simulink model "ADConverter_sim_2020"  (R2020b)
settings: Solver=ode4  StartTime=0.0  StopTime=20  FixedStep=0.05  RelTol=1e-3
settings Model: Creator=005274  LastModifiedBy=005274

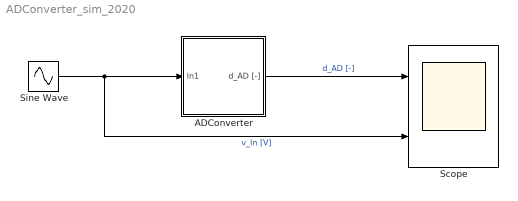
== system ADConverter_sim_2020 ==
  ADConverter : Subsystem  mask{n=10, V_max=5, V_min=0}
      mask prompts: n "Resolution : n bit"
  Scope : Scope  NumInputPorts=2
  Sine Wave : Sin  Amplitude=10  Frequency=2*pi*0.1  SampleTime=0
  wires:
  Sine Wave/1 -> Scope/2, ADConverter/1(In1)  "v_In [V]"
  ADConverter/1(d_AD [-]) -> Scope/1  "d_AD [-]"

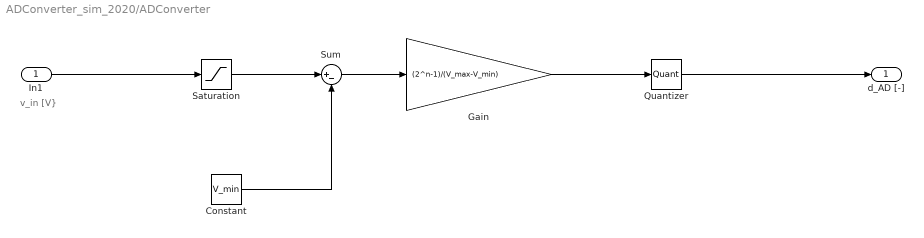
== system ADConverter_sim_2020/ADConverter ==
  note: v_in [V}
  In1 : Inport
  Constant : Constant  Value=V_min
  Gain : Gain  Gain=(2^n-1)/(V_max-V_min)
  Quantizer : Quantizer
  Saturation : Saturate  UpperLimit=V_max  LowerLimit=V_min
  Sum : Sum  Inputs=|+-
  d_AD [-] : Outport
  wires:
  In1/1 -> Saturation/1
  Gain/1 -> Quantizer/1
  Sum/1 -> Gain/1
  Saturation/1 -> Sum/1
  Quantizer/1 -> d_AD [-]/1
  Constant/1 -> Sum/2
